simulink model "W04_P0_plant"  (R2024b)
settings: Solver=ode4  StartTime=0.0  StopTime=10  FixedStep=0.001  RelTol=1e-3
values from neighbouring files (symbols this model uses):
  f_step = 1    [W04_setup.m]
  msd_b = 2    [W04_setup.m]
  msd_k = 2    [W04_setup.m]
  msd_m = 1    [W04_setup.m]
  plant_den = [1 2 2]    [W04_setup.m]
  plant_num = 1    [W04_setup.m]
settings Model: Creator=admin  LastModifiedBy=admin

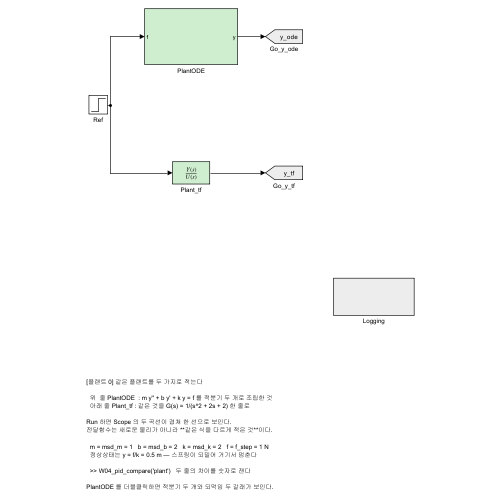
[thumbnail: Simulink's stored preview of the top-level diagram]
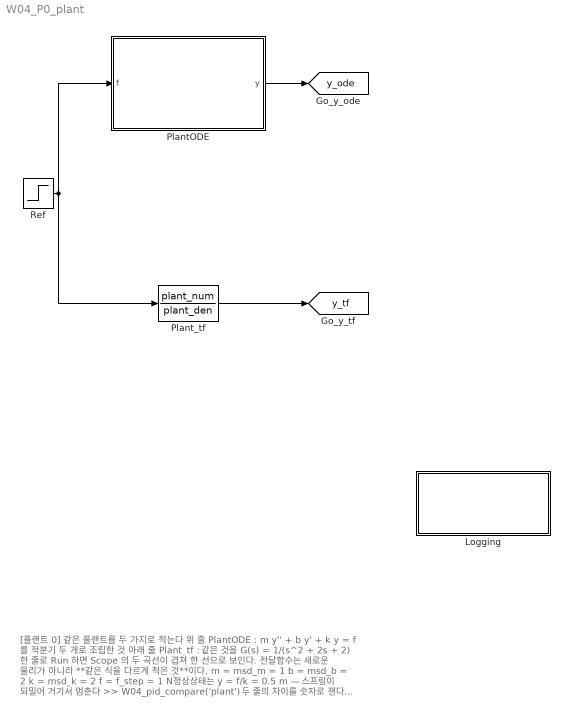
== system W04_P0_plant ==
  note: [플랜트 0] 같은 플랜트를 두 가지로 적는다
      |
      |   위  줄 PlantODE  : m y'' + b y' + k y = f 를 적분기 두 개로 조립한 것
      |   아래 줄 Plant_tf : 같은 것을 G(s) = 1/(s^2 + 2s + 2) 한 줄로
      |
      | Run 하면 Scope 의 두 곡선이 겹쳐 한 선으로 보인다.
      | 전달함수는 새로운 물리가 아니라 **같은 식을 다르게 적은 것**이다.
      |
      |   m = msd_m = 1   b = msd_b = 2   k = msd_k = 2   f = f_step = 1 N
      |   정상상태는 y = f/k = 0.5 m — 스프링이 되밀어 거기서 멈춘다
      |
      |   >> W04_pid_compare('plant')   두 줄의 차이를 숫자로 잰다
      |
      | PlantODE 를 더블클릭하면 적분기 두 개와 되먹임 두 갈래가 보인다.
  Logging : Subsystem
  PlantODE : Subsystem
  Plant_tf : TransferFcn  Numerator=plant_num  Denominator=plant_den
  Ref : Step  After=f_step  SampleTime=0
  tag scope: y_ode=global, y_tf=global
  wires:
  Ref/1 -> PlantODE/1(f), Plant_tf/1
  PlantODE/1(y) -> [y_ode]
  Plant_tf/1 -> [y_tf]

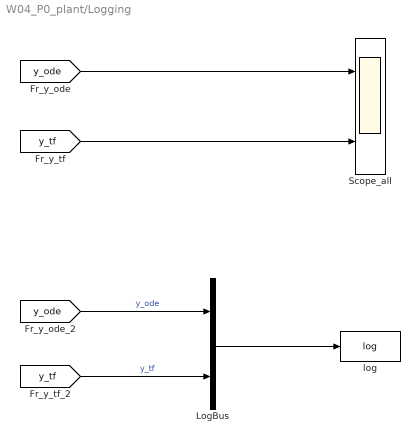
== system W04_P0_plant/Logging ==
  LogBus : BusCreator  Inputs=2
  Scope_all : Scope  NumInputPorts=2
  log : ToWorkspace  VariableName=log  SaveFormat=Timeseries  SampleTime=-1
  wires:
  [y_ode] -> Scope_all/1
  [y_tf] -> Scope_all/2
  [y_ode] -> LogBus/1  "y_ode"
  [y_tf] -> LogBus/2  "y_tf"
  LogBus/1 -> log/1

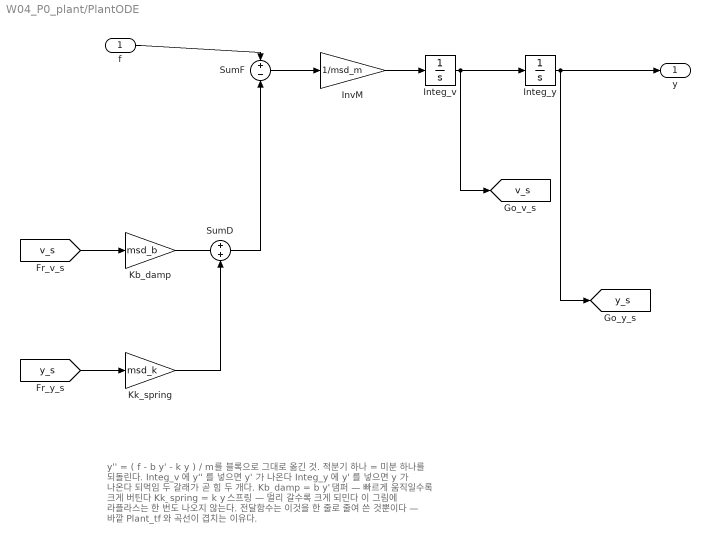
== system W04_P0_plant/PlantODE ==
  note: y'' = ( f - b y' - k y ) / m 를 블록으로 그대로 옮긴 것.
      |
      |   적분기 하나 = 미분 하나를 되돌린다.
      |     Integ_v 에 y'' 를 넣으면 y' 가 나온다
      |     Integ_y 에 y' 를 넣으면  y 가 나온다
      |
      |   되먹임 두 갈래가 곧 힘 두 개다.
      |     Kb_damp   = b y'   댐퍼 — 빠르게 움직일수록 크게 버틴다
      |     Kk_spring = k y    스프링 — 멀리 갈수록 크게 되민다
      |
      | 이 그림에 라플라스는 한 번도 나오지 않는다. 전달함수는 이것을
      | 한 줄로 줄여 쓴 것뿐이다 — 바깥 Plant_tf 와 곡선이 겹치는 이유다.
  f : Inport
  Integ_v : Integrator
  Integ_y : Integrator
  InvM : Gain  Gain=1/msd_m
  Kb_damp : Gain  Gain=msd_b
  Kk_spring : Gain  Gain=msd_k
  SumD : Sum
  SumF : Sum  Inputs=+-
  y : Outport
  tag scope: v_s=global, y_s=global
  wires:
  f/1 -> SumF/1
  SumF/1 -> InvM/1
  InvM/1 -> Integ_v/1
  Integ_v/1 -> Integ_y/1, [v_s]
  Integ_y/1 -> y/1, [y_s]
  [v_s] -> Kb_damp/1
  [y_s] -> Kk_spring/1
  Kb_damp/1 -> SumD/1
  Kk_spring/1 -> SumD/2
  SumD/1 -> SumF/2
